simulink model "AutomatedMBSE"  (R2020b)
settings: Solver=FixedStepAuto  StartTime=0.0  StopTime=60  FixedStep=5  RelTol=1e-3
undefined symbols (not defined in the file or in its folder): sigbuilder_block
settings Model: Creator=99003745  LastModifiedBy=99003745

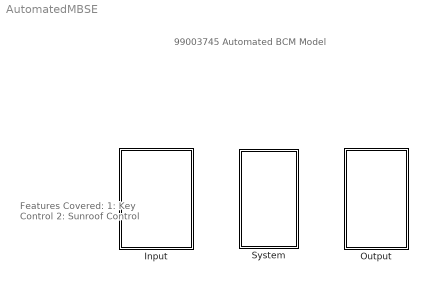
== system AutomatedMBSE ==
  note: Features Covered:
      | 1: Key Control
      | 2: Sunroof Control
  note: 99003745 Automated BCM Model
  Input : Subsystem
  Output : Subsystem
  System : Subsystem

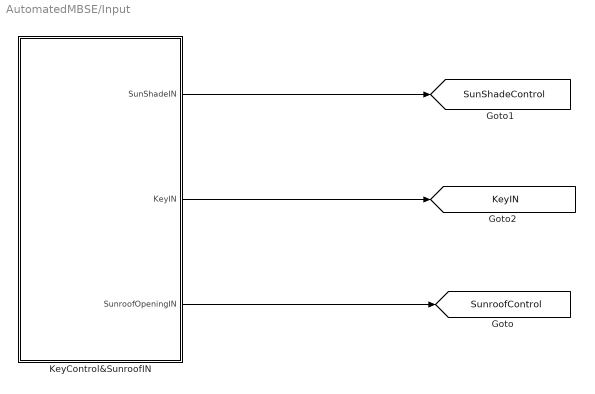
== system AutomatedMBSE/Input ==
  KeyControl&SunroofIN : Subsystem  Tag=STV Subsys  LoadFcn=sigbuilder_block('load',[558.75 205.5 550.5 399.75 ]);  StartFcn=sigbuilder_block('start');  StopFcn=sigbuilder_block('stop');  ClipboardFcn=sigbuilder_block('clipboard');  mask(Sigbuilder block){tuvar=[0:10]}
      mask help: Simulink:masks:SigbuilderBlock_MD
      mask init:
      | if ~strcmp(get_param(bdroot(gcbh),'SimulationStatus'),'stopped') tuvar = sigbuilder_block('maskInit'); end
      settings: CopyFcn=sigbuilder_block('copy');  DeleteFcn=sigbuilder_block('delete');  ModelCloseFcn=sigbuilder_block('modelClose');  PreSaveFcn=sigbuilder_block('preSave');  PauseFcn=sigbuilder_block('pause');  ContinueFcn=sigbuilder_block('continue');  NameChangeFcn=sigbuilder_block('namechange');  OpenFcn=sigbuilder_block('open',[558.75 205.5 550.5 399.75 ]);  CloseFcn=sigbuilder_block('close');
      mask Display: plot(0, 0, 100, 100,[2, 2, 32, 32, 2], [68, 8, 8, 68, 68],[32, 2], [38, 38], [32, 19, 2],[53, 60, 44], [32, 17, 17, 2],[16, 16, 31, 31]);txt = getActiveGroup(gcbh);text(2, 100, txt,'verticalAlignment', 'top');
  tag scope: KeyIN=global, SunShadeControl=global, SunroofControl=global
  wires:
  KeyControl&SunroofIN/2(KeyIN) -> [KeyIN]
  KeyControl&SunroofIN/1(SunShadeIN) -> [SunShadeControl]
  KeyControl&SunroofIN/3(SunroofOpeningIN) -> [SunroofControl]

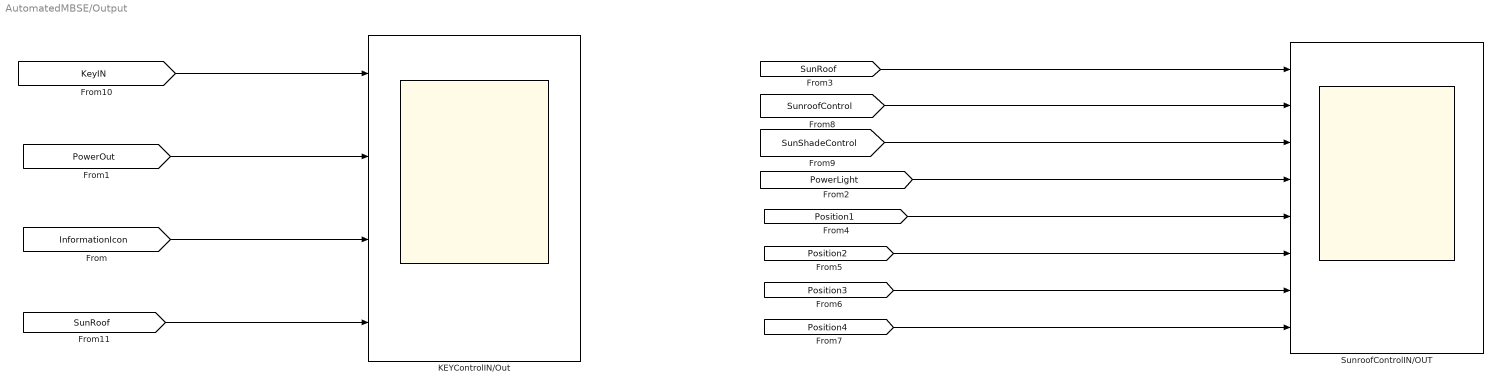
== system AutomatedMBSE/Output ==
  KEYControlIN/Out : Scope  NumInputPorts=4
  SunroofControlIN/OUT : Scope  NumInputPorts=8
  wires:
  [PowerOut] -> KEYControlIN/Out/2
  [InformationIcon] -> KEYControlIN/Out/3
  [SunRoof] -> SunroofControlIN/OUT/1
  [SunroofControl] -> SunroofControlIN/OUT/2
  [SunShadeControl] -> SunroofControlIN/OUT/3
  [PowerLight] -> SunroofControlIN/OUT/4
  [Position1] -> SunroofControlIN/OUT/5
  [Position2] -> SunroofControlIN/OUT/6
  [Position3] -> SunroofControlIN/OUT/7
  [Position4] -> SunroofControlIN/OUT/8
  [KeyIN] -> KEYControlIN/Out/1
  [SunRoof] -> KEYControlIN/Out/4

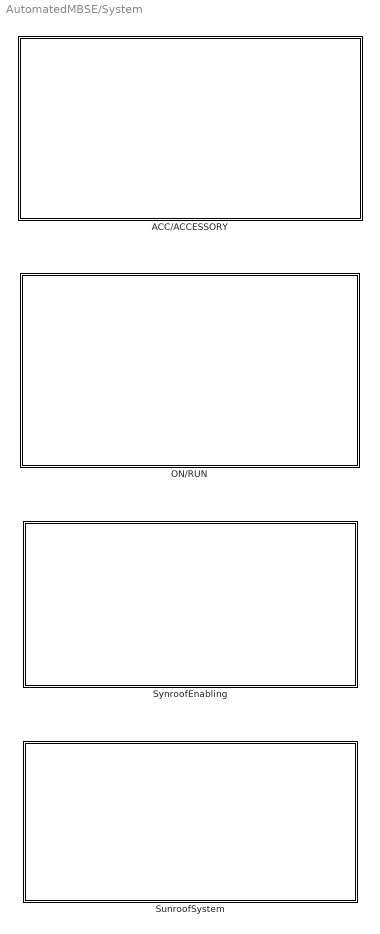
== system AutomatedMBSE/System ==
  ACC/ACCESSORY : Subsystem
  ON/RUN : Subsystem
  SunroofSystem : Subsystem
  SynroofEnabling : Subsystem

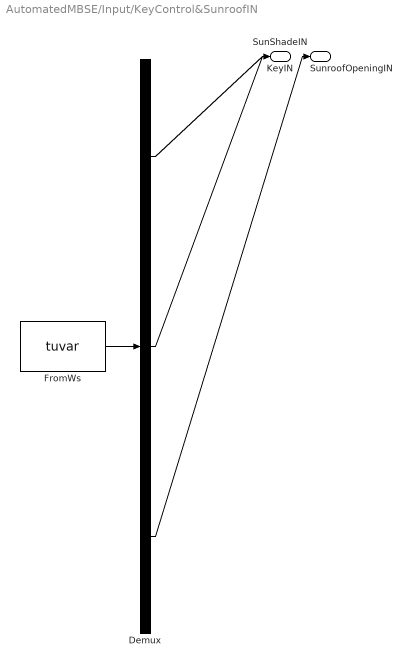
== system AutomatedMBSE/Input/KeyControl&SunroofIN ==
  Demux : Demux  Tag=STV Demux  Outputs=3
      settings: DisplayOption=none
  FromWs : FromWorkspace  Tag=STV FromWs  VariableName=tuvar
      SigBuilderData=|
      | common.afterFinalStr = 'Extrapolate'
      | common.sampleTime = 0
      | dataSet.timeRange = [0 60]
      | dataSet.name = 'Group 1'
      | sbobj.Groups.Name = 'Group 1'
      | sbobj.Groups.Signals(1).Name = 'SunShadeIN'
      | sbobj.Groups.Signals(1).XData = [0 2 4 6 8 10 12 14 16 18 20 22 24 26 28 30 32 34 36 38 40 42 44 46 48 50 52 54 56 58 60]
      | sbobj.Groups.Signals(1).YData = [0 0 0 0 0 -0.05 1 1 1 1 1 1 1 1 1 1 1 1 0 0 0 1 1 1 1 1 0 0 0 0 0]
      | sbobj.Groups.Signals(2).Name = 'KeyIN'
      | sbobj.Groups.Signals(2).XData = [0 2 4 6 8 10 12 14 16 18 20 22 24 26 28 30 32 34 36 38 40 42 44 46 48 50 52 54 56 58 60]
      | sbobj.Groups.Signals(2).YData = [0 0 0 0 1 1 1 1 2 2 2 2 3 3 3 3 2 2 2 2 1 1 1 1 0 0 0 0 0 1 1]
      | sbobj.Groups.Signals(3).Name = 'SunroofOpeningIN'
      | sbobj.Groups.Signals(3).XData = [0 2 4 6 8 10 12 14 16 18 20 22 24 26 28 30 32 34 36 38 40 42 44 46 48 50 52 54 56 58 60]
      | sbobj.Groups.Signals(3).YData = [0 10 20 30 40 50 60 70 80 90 100 90 80 70 60 50 40 30 20 10 0 10 20 30 40 50 60 70 80 90 100]
      | sbobj.Groups.TimeRange = [0 60]
  SunShadeIN : Outport  Tag=STV Outport
  KeyIN : Outport  Tag=STV Outport  Port=2
  SunroofOpeningIN : Outport  Tag=STV Outport  Port=3
  wires:
  FromWs/1 -> Demux/1
  Demux/1 -> SunShadeIN/1
  Demux/2 -> KeyIN/1
  Demux/3 -> SunroofOpeningIN/1

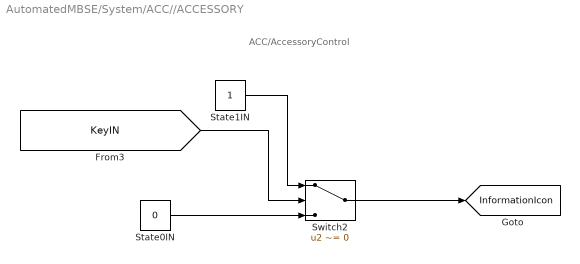
== system AutomatedMBSE/System/ACC//ACCESSORY ==
  note: ACC/AccessoryControl
  State0IN : Constant  Value=0
  State1IN : Constant
  Switch2 : Switch  Criteria=u2 ~= 0
  tag scope: InformationIcon=global
  wires:
  Switch2/1 -> [InformationIcon]
  [KeyIN] -> Switch2/2
  State0IN/1 -> Switch2/3
  State1IN/1 -> Switch2/1

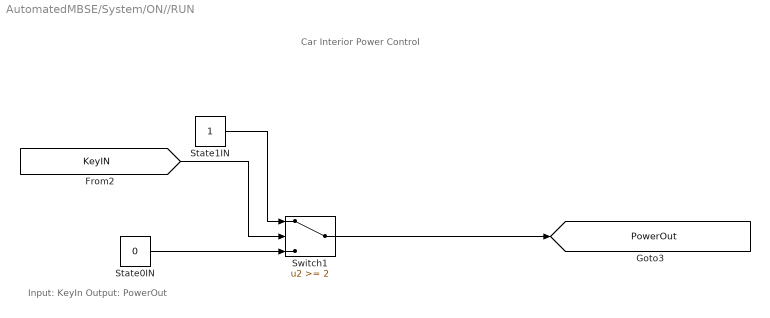
== system AutomatedMBSE/System/ON//RUN ==
  note: Input:
      | KeyIn
      | Output:
      | PowerOut
  note: Car Interior Power Control
  State0IN : Constant  Value=0
  State1IN : Constant
  Switch1 : Switch  Threshold=2
  tag scope: PowerOut=global
  wires:
  [KeyIN] -> Switch1/2
  Switch1/1 -> [PowerOut]
  State1IN/1 -> Switch1/1
  State0IN/1 -> Switch1/3

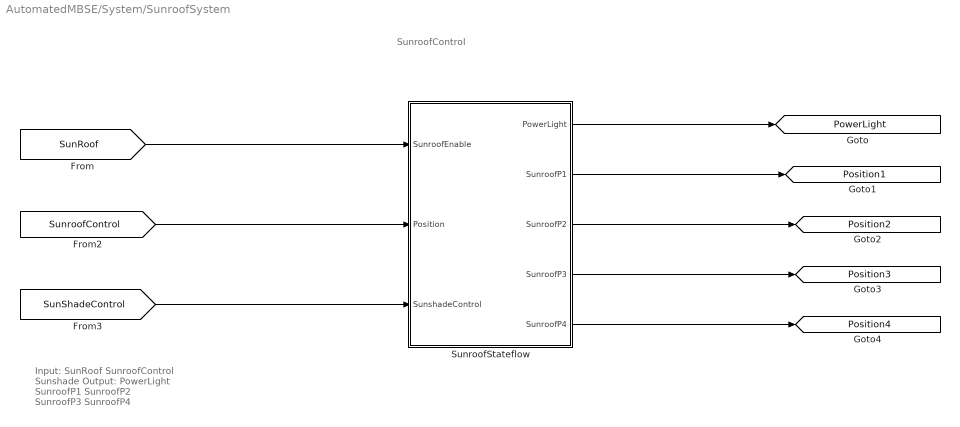
== system AutomatedMBSE/System/SunroofSystem ==
  note: Input:
      | SunRoof
      | SunroofControl
      | Sunshade
      | Output:
      | PowerLight
      | SunroofP1
      | SunroofP2
      | SunroofP3
      | SunroofP4
  note: SunroofControl
  SunroofStateflow : Stateflow chart  TreatAsAtomicUnit=on
  tag scope: Position1=global, Position2=global, Position3=global, Position4=global, PowerLight=global
  wires:
  [SunroofControl] -> SunroofStateflow/2(Position)
  [SunRoof] -> SunroofStateflow/1(SunroofEnable)
  [SunShadeControl] -> SunroofStateflow/3(SunshadeControl)
  SunroofStateflow/1(PowerLight) -> [PowerLight]
  SunroofStateflow/2(SunroofP1) -> [Position1]
  SunroofStateflow/3(SunroofP2) -> [Position2]
  SunroofStateflow/4(SunroofP3) -> [Position3]
  SunroofStateflow/5(SunroofP4) -> [Position4]

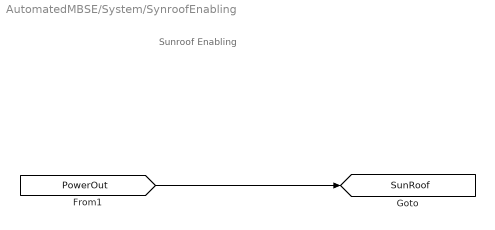
== system AutomatedMBSE/System/SynroofEnabling ==
  note: Sunroof Enabling
  tag scope: SunRoof=global
  wires:
  [PowerOut] -> [SunRoof]

== stateflow chart AutomatedMBSE/System/SunroofSystem/SunroofStateflow ==
  note: SunroofStateFlow
  state SunshadeOff
    entry:
    PowerLight=0;
  state SunshadeOn
    entry:
    PowerLight=1;
  state SunroofEnable
    entry:
    PowerLight=2;
    SunroofP1=0;
    SunroofP2=0;
    SunroofP3=0;
    SunroofP4=0;
  state P4
    entry:
    SunroofP1=1;
    SunroofP2=1;
    SunroofP3=1;
    SunroofP4=1;
  state P3
    entry:
    SunroofP1=1;
    SunroofP2=1;
    SunroofP3=1;
    SunroofP4=0;
  state P2
    entry:
    SunroofP1=1;
    SunroofP2=1;
    SunroofP3=0;
    SunroofP4=0;
  state P1
    entry:
    SunroofP1=1;
    SunroofP2=0;
    SunroofP3=0;
    SunroofP4=0;
  note: Input:
      | SunroofEnable
      | Position
      | SunshadeControl
      | Output:
      | PowerLight
      | SunroofP1
      | SunroofP2
      | SunroofP3
      | SunroofP4
  (default) -> SunshadeOff
  SunshadeOff -> SunshadeOn : [SunshadeControl==1]
  SunshadeOn -> SunshadeOff [order 2] : [SunshadeControl==0]
  SunroofEnable -> SunshadeOn [order 1] : [SunroofEnable==0]
  SunshadeOn -> SunroofEnable [order 1] : [SunshadeControl==1&&SunroofEnable==1]
  P4 -> SunroofEnable [order 2] : [SunshadeControl==0&&SunroofEnable==0]
  SunroofEnable -> P3 [order 4] : [SunshadeControl==1&&SunroofEnable==1 && Position>=50 && Position<=75]
  SunroofEnable -> P4 [order 3] : [SunshadeControl==1&&SunroofEnable==1 && Position>75 && Position<=100]
  SunroofEnable -> P1 [order 2] : [SunshadeControl==1&&SunroofEnable==1 && Position>0 && Position<=25]
  P3 -> SunroofEnable [order 3] : [SunshadeControl==0&&SunroofEnable==0]
  P1 -> SunroofEnable [order 2] : [SunshadeControl==0&&SunroofEnable==0 && Position>=0 && Position<50]
  P2 -> SunroofEnable [order 3] : [SunshadeControl==0&&SunroofEnable==0]
  SunroofEnable -> P2 [order 5] : [SunshadeControl==1&&SunroofEnable==1 && Position>=25 && Position<50]
  P1 -> P2 [order 1] : [SunshadeControl==1&&SunroofEnable==1 && Position>=25 && Position<50]
  P2 -> P3 [order 1] : [SunshadeControl==1&&SunroofEnable==1 && Position>=50 && Position<75]
  P3 -> P4 [order 1] : [SunshadeControl==1&&SunroofEnable==1 && Position>=75 && Position<100]
  P2 -> P1 [order 2] : [SunshadeControl==1&&SunroofEnable==1 && Position>0 && Position<=25]
  P3 -> P2 [order 2] : [SunshadeControl==1&&SunroofEnable==1 && Position>25&& Position<=50]
  P4 -> P3 [order 1] : [SunshadeControl==1&&SunroofEnable==1 && Position>50 && Position<=75]
  data: SunroofEnable input; Position input; SunshadeControl input; PowerLight output; SunroofP1 output; SunroofP2 output; SunroofP3 output; SunroofP4 output
